simulink model "AVIC_model"  (R2015b)
settings: Solver=ode45  StartTime=0.0  StopTime=simtime  RelTol=1e-3
values from neighbouring files (symbols this model uses):
  A = 1    [simulation.m]
  a1 = 1    [simulation.m]
  a2 = 3    [simulation.m]
  a3 = 3    [simulation.m]
  Amp1 = Ampl/1000000    (= 134.217728)    [simulation.m]
  b1 = 1    [simulation.m]
  B2 = 8    [simulation.m]
  C = 32    [simulation.m]
  c1 = 1    [simulation.m]
  c2 = 1    [simulation.m]
  c3 = 1    [simulation.m]
  finrad = 2*pi/(N)*f0*clk    [simulation.m]
  FSC = 2^27    (= 134217728)    [simulation.m]
  SAT = 127    [simulation.m]
  Ts = 1/clk    (= 1.62760416667e-07)    [simulation.m]
libraries: simulink x298
(part 3 of 5)

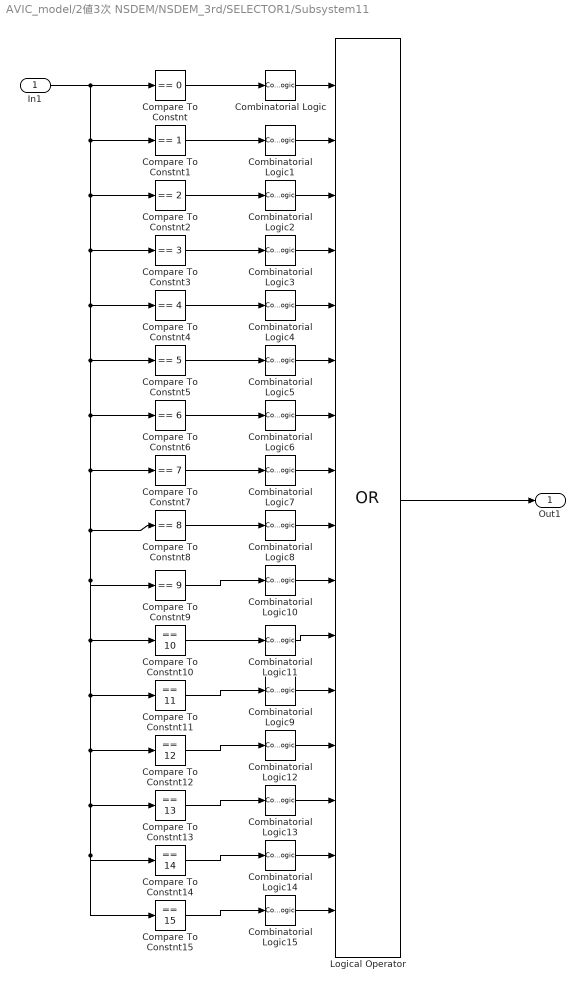
== system AVIC_model/2値3次 NSDEM/NSDEM_3rd/SELECTOR1/Subsystem11 ==
  In1 : Inport
  Combinatorial Logic : CombinatorialLogic  TruthTable=[0 0 0 0 0 0 0 0 0 0 0 0 0 0 0 0;1 0 0 0 0 0 0 0 0 0 0 0 0 0 0 0]
  Combinatorial Logic1 : CombinatorialLogic  TruthTable=[0 0 0 0 0 0 0 0 0 0 0 0 0 0 0 0; 0 1 0 0 0 0 0 0 0 0 0 0 0 0 0 0]
  Combinatorial Logic10 : CombinatorialLogic  TruthTable=[0 0 0 0 0 0 0 0 0 0 0 0 0 0 0 0;0 0 0 0 0 0 0 0 0 1 0 0 0 0 0 0]
  Combinatorial Logic11 : CombinatorialLogic  TruthTable=[0 0 0 0 0 0 0 0 0 0 0 0 0 0 0 0;0 0 0 0 0 0 0 0 0 0 1 0 0 0 0 0 ]
  Combinatorial Logic12 : CombinatorialLogic  TruthTable=[0 0 0 0 0 0 0 0 0 0 0 0 0 0 0 0;0 0 0 0 0 0 0 0 0 0 0 0 1 0 0 0]
  Combinatorial Logic13 : CombinatorialLogic  TruthTable=[0 0 0 0 0 0 0 0 0 0 0 0 0 0 0 0;0 0 0 0 0 0 0 0 0 0 0 0 0 1 0 0]
  Combinatorial Logic14 : CombinatorialLogic  TruthTable=[0 0 0 0 0 0 0 0 0 0 0 0 0 0 0 0;0 0 0 0 0 0 0 0 0 0 0 0 0 0 1 0]
  Combinatorial Logic15 : CombinatorialLogic  TruthTable=[0 0 0 0 0 0 0 0 0 0 0 0 0 0 0 0;0 0 0 0 0 0 0 0 0 0 0 0 0 0 0 1]
  Combinatorial Logic2 : CombinatorialLogic  TruthTable=[0 0 0 0 0 0 0 0 0 0 0 0 0 0 0 0;0 0 1 0 0 0 0 0 0 0 0 0 0 0 0 0]
  Combinatorial Logic3 : CombinatorialLogic  TruthTable=[0 0 0 0 0 0 0 0 0 0 0 0 0 0 0 0;0 0 0 1 0 0 0 0 0 0 0 0 0 0 0 0]
  Combinatorial Logic4 : CombinatorialLogic  TruthTable=[0 0 0 0 0 0 0 0 0 0 0 0 0 0 0 0;0 0 0 0 1 0 0 0 0 0 0 0 0 0 0 0]
  Combinatorial Logic5 : CombinatorialLogic  TruthTable=[0 0 0 0 0 0 0 0 0 0 0 0 0 0 0 0;0 0 0 0 0 1 0 0 0 0 0 0 0 0 0 0]
  Combinatorial Logic6 : CombinatorialLogic  TruthTable=[0 0 0 0 0 0 0 0 0 0 0 0 0 0 0 0;0 0 0 0 0 0 1 0 0 0 0 0 0 0 0 0]
  Combinatorial Logic7 : CombinatorialLogic  TruthTable=[0 0 0 0 0 0 0 0 0 0 0 0 0 0 0 0;0 0 0 0 0 0 0 1 0 0 0 0 0 0 0 0]
  Combinatorial Logic8 : CombinatorialLogic  TruthTable=[0 0 0 0 0 0 0 0 0 0 0 0 0 0 0 0;0 0 0 0 0 0 0 0 1 0 0 0 0 0 0 0]
  Combinatorial Logic9 : CombinatorialLogic  TruthTable=[0 0 0 0 0 0 0 0 0 0 0 0 0 0 0 0;0 0 0 0 0 0 0 0 0 0 0 1 0 0 0 0 ]
  Compare To Constnt : simulink/Logic and Bit Operations/Compare To Constant  relop===  const=0  OutDataTypeStr=boolean  ZeroCross=off
  Compare To Constnt1 : simulink/Logic and Bit Operations/Compare To Constant  relop===  const=1  OutDataTypeStr=boolean  ZeroCross=off
  Compare To Constnt10 : simulink/Logic and Bit Operations/Compare To Constant  relop===  const=10  OutDataTypeStr=boolean  ZeroCross=off
  Compare To Constnt11 : simulink/Logic and Bit Operations/Compare To Constant  relop===  const=11  OutDataTypeStr=boolean  ZeroCross=off
  Compare To Constnt12 : simulink/Logic and Bit Operations/Compare To Constant  relop===  const=12  OutDataTypeStr=boolean  ZeroCross=off
  Compare To Constnt13 : simulink/Logic and Bit Operations/Compare To Constant  relop===  const=13  OutDataTypeStr=boolean  ZeroCross=off
  Compare To Constnt14 : simulink/Logic and Bit Operations/Compare To Constant  relop===  const=14  OutDataTypeStr=boolean  ZeroCross=off
  Compare To Constnt15 : simulink/Logic and Bit Operations/Compare To Constant  relop===  const=15  OutDataTypeStr=boolean  ZeroCross=off
  Compare To Constnt2 : simulink/Logic and Bit Operations/Compare To Constant  relop===  const=2  OutDataTypeStr=boolean  ZeroCross=off
  Compare To Constnt3 : simulink/Logic and Bit Operations/Compare To Constant  relop===  const=3  OutDataTypeStr=boolean  ZeroCross=off
  Compare To Constnt4 : simulink/Logic and Bit Operations/Compare To Constant  relop===  const=4  OutDataTypeStr=boolean  ZeroCross=off
  Compare To Constnt5 : simulink/Logic and Bit Operations/Compare To Constant  relop===  const=5  OutDataTypeStr=boolean  ZeroCross=off
  Compare To Constnt6 : simulink/Logic and Bit Operations/Compare To Constant  relop===  const=6  OutDataTypeStr=boolean  ZeroCross=off
  Compare To Constnt7 : simulink/Logic and Bit Operations/Compare To Constant  relop===  const=7  OutDataTypeStr=boolean  ZeroCross=off
  Compare To Constnt8 : simulink/Logic and Bit Operations/Compare To Constant  relop===  const=8  OutDataTypeStr=boolean  ZeroCross=off
  Compare To Constnt9 : simulink/Logic and Bit Operations/Compare To Constant  relop===  const=9  OutDataTypeStr=boolean  ZeroCross=off
  Logical Operator : Logic  Operator=OR  Inputs=16  AllPortsSameDT=off  OutDataTypeStr=boolean
  Out1 : Outport
  wires:
  Logical Operator/1 -> Out1/1
  In1/1 -> Compare To Constnt/1, Compare To Constnt1/1, Compare To Constnt2/1, Compare To Constnt3/1, Compare To Constnt4/1, Compare To Constnt5/1, Compare To Constnt6/1, Compare To Constnt7/1, Compare To Constnt8/1, Compare To Constnt9/1, Compare To Constnt10/1, Compare To Constnt11/1, Compare To Constnt12/1, Compare To Constnt13/1, Compare To Constnt15/1, Compare To Constnt14/1
  Compare To Constnt/1 -> Combinatorial Logic/1
  Compare To Constnt1/1 -> Combinatorial Logic1/1
  Compare To Constnt2/1 -> Combinatorial Logic2/1
  Compare To Constnt3/1 -> Combinatorial Logic3/1
  Compare To Constnt4/1 -> Combinatorial Logic4/1
  Compare To Constnt5/1 -> Combinatorial Logic5/1
  Compare To Constnt6/1 -> Combinatorial Logic6/1
  Compare To Constnt7/1 -> Combinatorial Logic7/1
  Combinatorial Logic/1 -> Logical Operator/1
  Combinatorial Logic1/1 -> Logical Operator/2
  Combinatorial Logic2/1 -> Logical Operator/3
  Combinatorial Logic3/1 -> Logical Operator/4
  Combinatorial Logic4/1 -> Logical Operator/5
  Combinatorial Logic5/1 -> Logical Operator/6
  Combinatorial Logic6/1 -> Logical Operator/7
  Combinatorial Logic7/1 -> Logical Operator/8
  Compare To Constnt8/1 -> Combinatorial Logic8/1
  Compare To Constnt9/1 -> Combinatorial Logic10/1
  Compare To Constnt10/1 -> Combinatorial Logic11/1
  Compare To Constnt11/1 -> Combinatorial Logic9/1
  Compare To Constnt12/1 -> Combinatorial Logic12/1
  Compare To Constnt13/1 -> Combinatorial Logic13/1
  Compare To Constnt14/1 -> Combinatorial Logic14/1
  Compare To Constnt15/1 -> Combinatorial Logic15/1
  Combinatorial Logic8/1 -> Logical Operator/9
  Combinatorial Logic10/1 -> Logical Operator/10
  Combinatorial Logic11/1 -> Logical Operator/11
  Combinatorial Logic9/1 -> Logical Operator/12
  Combinatorial Logic12/1 -> Logical Operator/13
  Combinatorial Logic13/1 -> Logical Operator/14
  Combinatorial Logic14/1 -> Logical Operator/15
  Combinatorial Logic15/1 -> Logical Operator/16

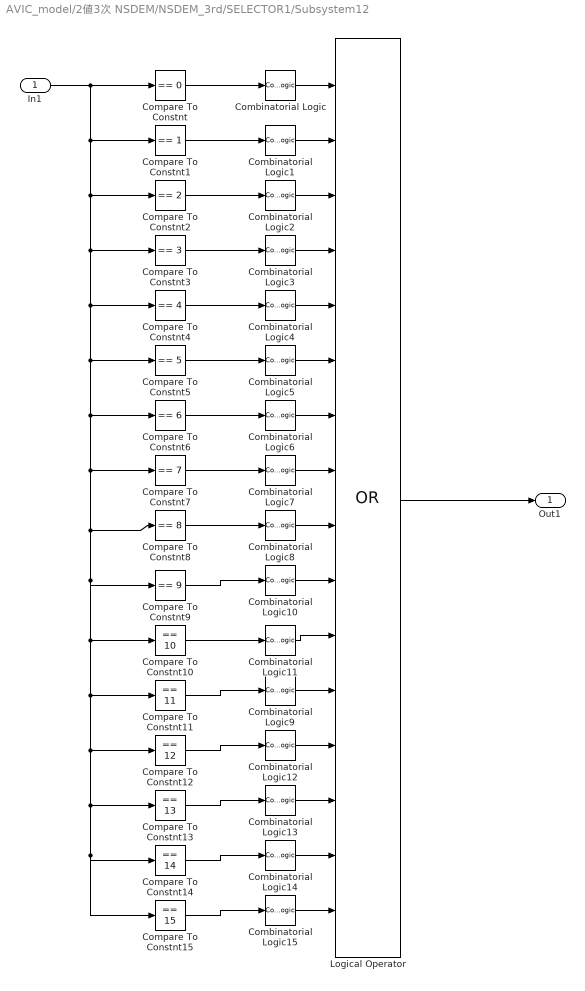
== system AVIC_model/2値3次 NSDEM/NSDEM_3rd/SELECTOR1/Subsystem12 ==
  In1 : Inport
  Combinatorial Logic : CombinatorialLogic  TruthTable=[0 0 0 0 0 0 0 0 0 0 0 0 0 0 0 0;1 0 0 0 0 0 0 0 0 0 0 0 0 0 0 0]
  Combinatorial Logic1 : CombinatorialLogic  TruthTable=[0 0 0 0 0 0 0 0 0 0 0 0 0 0 0 0; 0 1 0 0 0 0 0 0 0 0 0 0 0 0 0 0]
  Combinatorial Logic10 : CombinatorialLogic  TruthTable=[0 0 0 0 0 0 0 0 0 0 0 0 0 0 0 0;0 0 0 0 0 0 0 0 0 1 0 0 0 0 0 0]
  Combinatorial Logic11 : CombinatorialLogic  TruthTable=[0 0 0 0 0 0 0 0 0 0 0 0 0 0 0 0;0 0 0 0 0 0 0 0 0 0 1 0 0 0 0 0 ]
  Combinatorial Logic12 : CombinatorialLogic  TruthTable=[0 0 0 0 0 0 0 0 0 0 0 0 0 0 0 0;0 0 0 0 0 0 0 0 0 0 0 0 1 0 0 0]
  Combinatorial Logic13 : CombinatorialLogic  TruthTable=[0 0 0 0 0 0 0 0 0 0 0 0 0 0 0 0;0 0 0 0 0 0 0 0 0 0 0 0 0 1 0 0]
  Combinatorial Logic14 : CombinatorialLogic  TruthTable=[0 0 0 0 0 0 0 0 0 0 0 0 0 0 0 0;0 0 0 0 0 0 0 0 0 0 0 0 0 0 1 0]
  Combinatorial Logic15 : CombinatorialLogic  TruthTable=[0 0 0 0 0 0 0 0 0 0 0 0 0 0 0 0;0 0 0 0 0 0 0 0 0 0 0 0 0 0 0 1]
  Combinatorial Logic2 : CombinatorialLogic  TruthTable=[0 0 0 0 0 0 0 0 0 0 0 0 0 0 0 0;0 0 1 0 0 0 0 0 0 0 0 0 0 0 0 0]
  Combinatorial Logic3 : CombinatorialLogic  TruthTable=[0 0 0 0 0 0 0 0 0 0 0 0 0 0 0 0;0 0 0 1 0 0 0 0 0 0 0 0 0 0 0 0]
  Combinatorial Logic4 : CombinatorialLogic  TruthTable=[0 0 0 0 0 0 0 0 0 0 0 0 0 0 0 0;0 0 0 0 1 0 0 0 0 0 0 0 0 0 0 0]
  Combinatorial Logic5 : CombinatorialLogic  TruthTable=[0 0 0 0 0 0 0 0 0 0 0 0 0 0 0 0;0 0 0 0 0 1 0 0 0 0 0 0 0 0 0 0]
  Combinatorial Logic6 : CombinatorialLogic  TruthTable=[0 0 0 0 0 0 0 0 0 0 0 0 0 0 0 0;0 0 0 0 0 0 1 0 0 0 0 0 0 0 0 0]
  Combinatorial Logic7 : CombinatorialLogic  TruthTable=[0 0 0 0 0 0 0 0 0 0 0 0 0 0 0 0;0 0 0 0 0 0 0 1 0 0 0 0 0 0 0 0]
  Combinatorial Logic8 : CombinatorialLogic  TruthTable=[0 0 0 0 0 0 0 0 0 0 0 0 0 0 0 0;0 0 0 0 0 0 0 0 1 0 0 0 0 0 0 0]
  Combinatorial Logic9 : CombinatorialLogic  TruthTable=[0 0 0 0 0 0 0 0 0 0 0 0 0 0 0 0;0 0 0 0 0 0 0 0 0 0 0 1 0 0 0 0 ]
  Compare To Constnt : simulink/Logic and Bit Operations/Compare To Constant  relop===  const=0  OutDataTypeStr=boolean  ZeroCross=off
  Compare To Constnt1 : simulink/Logic and Bit Operations/Compare To Constant  relop===  const=1  OutDataTypeStr=boolean  ZeroCross=off
  Compare To Constnt10 : simulink/Logic and Bit Operations/Compare To Constant  relop===  const=10  OutDataTypeStr=boolean  ZeroCross=off
  Compare To Constnt11 : simulink/Logic and Bit Operations/Compare To Constant  relop===  const=11  OutDataTypeStr=boolean  ZeroCross=off
  Compare To Constnt12 : simulink/Logic and Bit Operations/Compare To Constant  relop===  const=12  OutDataTypeStr=boolean  ZeroCross=off
  Compare To Constnt13 : simulink/Logic and Bit Operations/Compare To Constant  relop===  const=13  OutDataTypeStr=boolean  ZeroCross=off
  Compare To Constnt14 : simulink/Logic and Bit Operations/Compare To Constant  relop===  const=14  OutDataTypeStr=boolean  ZeroCross=off
  Compare To Constnt15 : simulink/Logic and Bit Operations/Compare To Constant  relop===  const=15  OutDataTypeStr=boolean  ZeroCross=off
  Compare To Constnt2 : simulink/Logic and Bit Operations/Compare To Constant  relop===  const=2  OutDataTypeStr=boolean  ZeroCross=off
  Compare To Constnt3 : simulink/Logic and Bit Operations/Compare To Constant  relop===  const=3  OutDataTypeStr=boolean  ZeroCross=off
  Compare To Constnt4 : simulink/Logic and Bit Operations/Compare To Constant  relop===  const=4  OutDataTypeStr=boolean  ZeroCross=off
  Compare To Constnt5 : simulink/Logic and Bit Operations/Compare To Constant  relop===  const=5  OutDataTypeStr=boolean  ZeroCross=off
  Compare To Constnt6 : simulink/Logic and Bit Operations/Compare To Constant  relop===  const=6  OutDataTypeStr=boolean  ZeroCross=off
  Compare To Constnt7 : simulink/Logic and Bit Operations/Compare To Constant  relop===  const=7  OutDataTypeStr=boolean  ZeroCross=off
  Compare To Constnt8 : simulink/Logic and Bit Operations/Compare To Constant  relop===  const=8  OutDataTypeStr=boolean  ZeroCross=off
  Compare To Constnt9 : simulink/Logic and Bit Operations/Compare To Constant  relop===  const=9  OutDataTypeStr=boolean  ZeroCross=off
  Logical Operator : Logic  Operator=OR  Inputs=16  AllPortsSameDT=off  OutDataTypeStr=boolean
  Out1 : Outport
  wires:
  Logical Operator/1 -> Out1/1
  In1/1 -> Compare To Constnt/1, Compare To Constnt1/1, Compare To Constnt2/1, Compare To Constnt3/1, Compare To Constnt4/1, Compare To Constnt5/1, Compare To Constnt6/1, Compare To Constnt7/1, Compare To Constnt8/1, Compare To Constnt9/1, Compare To Constnt10/1, Compare To Constnt11/1, Compare To Constnt12/1, Compare To Constnt13/1, Compare To Constnt15/1, Compare To Constnt14/1
  Compare To Constnt/1 -> Combinatorial Logic/1
  Compare To Constnt1/1 -> Combinatorial Logic1/1
  Compare To Constnt2/1 -> Combinatorial Logic2/1
  Compare To Constnt3/1 -> Combinatorial Logic3/1
  Compare To Constnt4/1 -> Combinatorial Logic4/1
  Compare To Constnt5/1 -> Combinatorial Logic5/1
  Compare To Constnt6/1 -> Combinatorial Logic6/1
  Compare To Constnt7/1 -> Combinatorial Logic7/1
  Combinatorial Logic/1 -> Logical Operator/1
  Combinatorial Logic1/1 -> Logical Operator/2
  Combinatorial Logic2/1 -> Logical Operator/3
  Combinatorial Logic3/1 -> Logical Operator/4
  Combinatorial Logic4/1 -> Logical Operator/5
  Combinatorial Logic5/1 -> Logical Operator/6
  Combinatorial Logic6/1 -> Logical Operator/7
  Combinatorial Logic7/1 -> Logical Operator/8
  Compare To Constnt8/1 -> Combinatorial Logic8/1
  Compare To Constnt9/1 -> Combinatorial Logic10/1
  Compare To Constnt10/1 -> Combinatorial Logic11/1
  Compare To Constnt11/1 -> Combinatorial Logic9/1
  Compare To Constnt12/1 -> Combinatorial Logic12/1
  Compare To Constnt13/1 -> Combinatorial Logic13/1
  Compare To Constnt14/1 -> Combinatorial Logic14/1
  Compare To Constnt15/1 -> Combinatorial Logic15/1
  Combinatorial Logic8/1 -> Logical Operator/9
  Combinatorial Logic10/1 -> Logical Operator/10
  Combinatorial Logic11/1 -> Logical Operator/11
  Combinatorial Logic9/1 -> Logical Operator/12
  Combinatorial Logic12/1 -> Logical Operator/13
  Combinatorial Logic13/1 -> Logical Operator/14
  Combinatorial Logic14/1 -> Logical Operator/15
  Combinatorial Logic15/1 -> Logical Operator/16

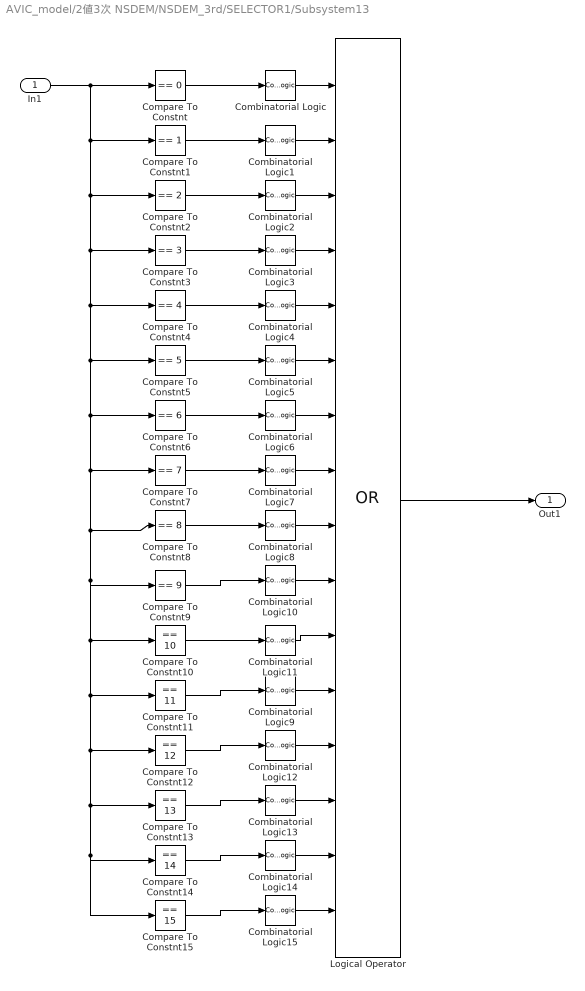
== system AVIC_model/2値3次 NSDEM/NSDEM_3rd/SELECTOR1/Subsystem13 ==
  In1 : Inport
  Combinatorial Logic : CombinatorialLogic  TruthTable=[0 0 0 0 0 0 0 0 0 0 0 0 0 0 0 0;1 0 0 0 0 0 0 0 0 0 0 0 0 0 0 0]
  Combinatorial Logic1 : CombinatorialLogic  TruthTable=[0 0 0 0 0 0 0 0 0 0 0 0 0 0 0 0; 0 1 0 0 0 0 0 0 0 0 0 0 0 0 0 0]
  Combinatorial Logic10 : CombinatorialLogic  TruthTable=[0 0 0 0 0 0 0 0 0 0 0 0 0 0 0 0;0 0 0 0 0 0 0 0 0 1 0 0 0 0 0 0]
  Combinatorial Logic11 : CombinatorialLogic  TruthTable=[0 0 0 0 0 0 0 0 0 0 0 0 0 0 0 0;0 0 0 0 0 0 0 0 0 0 1 0 0 0 0 0 ]
  Combinatorial Logic12 : CombinatorialLogic  TruthTable=[0 0 0 0 0 0 0 0 0 0 0 0 0 0 0 0;0 0 0 0 0 0 0 0 0 0 0 0 1 0 0 0]
  Combinatorial Logic13 : CombinatorialLogic  TruthTable=[0 0 0 0 0 0 0 0 0 0 0 0 0 0 0 0;0 0 0 0 0 0 0 0 0 0 0 0 0 1 0 0]
  Combinatorial Logic14 : CombinatorialLogic  TruthTable=[0 0 0 0 0 0 0 0 0 0 0 0 0 0 0 0;0 0 0 0 0 0 0 0 0 0 0 0 0 0 1 0]
  Combinatorial Logic15 : CombinatorialLogic  TruthTable=[0 0 0 0 0 0 0 0 0 0 0 0 0 0 0 0;0 0 0 0 0 0 0 0 0 0 0 0 0 0 0 1]
  Combinatorial Logic2 : CombinatorialLogic  TruthTable=[0 0 0 0 0 0 0 0 0 0 0 0 0 0 0 0;0 0 1 0 0 0 0 0 0 0 0 0 0 0 0 0]
  Combinatorial Logic3 : CombinatorialLogic  TruthTable=[0 0 0 0 0 0 0 0 0 0 0 0 0 0 0 0;0 0 0 1 0 0 0 0 0 0 0 0 0 0 0 0]
  Combinatorial Logic4 : CombinatorialLogic  TruthTable=[0 0 0 0 0 0 0 0 0 0 0 0 0 0 0 0;0 0 0 0 1 0 0 0 0 0 0 0 0 0 0 0]
  Combinatorial Logic5 : CombinatorialLogic  TruthTable=[0 0 0 0 0 0 0 0 0 0 0 0 0 0 0 0;0 0 0 0 0 1 0 0 0 0 0 0 0 0 0 0]
  Combinatorial Logic6 : CombinatorialLogic  TruthTable=[0 0 0 0 0 0 0 0 0 0 0 0 0 0 0 0;0 0 0 0 0 0 1 0 0 0 0 0 0 0 0 0]
  Combinatorial Logic7 : CombinatorialLogic  TruthTable=[0 0 0 0 0 0 0 0 0 0 0 0 0 0 0 0;0 0 0 0 0 0 0 1 0 0 0 0 0 0 0 0]
  Combinatorial Logic8 : CombinatorialLogic  TruthTable=[0 0 0 0 0 0 0 0 0 0 0 0 0 0 0 0;0 0 0 0 0 0 0 0 1 0 0 0 0 0 0 0]
  Combinatorial Logic9 : CombinatorialLogic  TruthTable=[0 0 0 0 0 0 0 0 0 0 0 0 0 0 0 0;0 0 0 0 0 0 0 0 0 0 0 1 0 0 0 0 ]
  Compare To Constnt : simulink/Logic and Bit Operations/Compare To Constant  relop===  const=0  OutDataTypeStr=boolean  ZeroCross=off
  Compare To Constnt1 : simulink/Logic and Bit Operations/Compare To Constant  relop===  const=1  OutDataTypeStr=boolean  ZeroCross=off
  Compare To Constnt10 : simulink/Logic and Bit Operations/Compare To Constant  relop===  const=10  OutDataTypeStr=boolean  ZeroCross=off
  Compare To Constnt11 : simulink/Logic and Bit Operations/Compare To Constant  relop===  const=11  OutDataTypeStr=boolean  ZeroCross=off
  Compare To Constnt12 : simulink/Logic and Bit Operations/Compare To Constant  relop===  const=12  OutDataTypeStr=boolean  ZeroCross=off
  Compare To Constnt13 : simulink/Logic and Bit Operations/Compare To Constant  relop===  const=13  OutDataTypeStr=boolean  ZeroCross=off
  Compare To Constnt14 : simulink/Logic and Bit Operations/Compare To Constant  relop===  const=14  OutDataTypeStr=boolean  ZeroCross=off
  Compare To Constnt15 : simulink/Logic and Bit Operations/Compare To Constant  relop===  const=15  OutDataTypeStr=boolean  ZeroCross=off
  Compare To Constnt2 : simulink/Logic and Bit Operations/Compare To Constant  relop===  const=2  OutDataTypeStr=boolean  ZeroCross=off
  Compare To Constnt3 : simulink/Logic and Bit Operations/Compare To Constant  relop===  const=3  OutDataTypeStr=boolean  ZeroCross=off
  Compare To Constnt4 : simulink/Logic and Bit Operations/Compare To Constant  relop===  const=4  OutDataTypeStr=boolean  ZeroCross=off
  Compare To Constnt5 : simulink/Logic and Bit Operations/Compare To Constant  relop===  const=5  OutDataTypeStr=boolean  ZeroCross=off
  Compare To Constnt6 : simulink/Logic and Bit Operations/Compare To Constant  relop===  const=6  OutDataTypeStr=boolean  ZeroCross=off
  Compare To Constnt7 : simulink/Logic and Bit Operations/Compare To Constant  relop===  const=7  OutDataTypeStr=boolean  ZeroCross=off
  Compare To Constnt8 : simulink/Logic and Bit Operations/Compare To Constant  relop===  const=8  OutDataTypeStr=boolean  ZeroCross=off
  Compare To Constnt9 : simulink/Logic and Bit Operations/Compare To Constant  relop===  const=9  OutDataTypeStr=boolean  ZeroCross=off
  Logical Operator : Logic  Operator=OR  Inputs=16  AllPortsSameDT=off  OutDataTypeStr=boolean
  Out1 : Outport
  wires:
  Logical Operator/1 -> Out1/1
  In1/1 -> Compare To Constnt/1, Compare To Constnt1/1, Compare To Constnt2/1, Compare To Constnt3/1, Compare To Constnt4/1, Compare To Constnt5/1, Compare To Constnt6/1, Compare To Constnt7/1, Compare To Constnt8/1, Compare To Constnt9/1, Compare To Constnt10/1, Compare To Constnt11/1, Compare To Constnt12/1, Compare To Constnt13/1, Compare To Constnt15/1, Compare To Constnt14/1
  Compare To Constnt/1 -> Combinatorial Logic/1
  Compare To Constnt1/1 -> Combinatorial Logic1/1
  Compare To Constnt2/1 -> Combinatorial Logic2/1
  Compare To Constnt3/1 -> Combinatorial Logic3/1
  Compare To Constnt4/1 -> Combinatorial Logic4/1
  Compare To Constnt5/1 -> Combinatorial Logic5/1
  Compare To Constnt6/1 -> Combinatorial Logic6/1
  Compare To Constnt7/1 -> Combinatorial Logic7/1
  Combinatorial Logic/1 -> Logical Operator/1
  Combinatorial Logic1/1 -> Logical Operator/2
  Combinatorial Logic2/1 -> Logical Operator/3
  Combinatorial Logic3/1 -> Logical Operator/4
  Combinatorial Logic4/1 -> Logical Operator/5
  Combinatorial Logic5/1 -> Logical Operator/6
  Combinatorial Logic6/1 -> Logical Operator/7
  Combinatorial Logic7/1 -> Logical Operator/8
  Compare To Constnt8/1 -> Combinatorial Logic8/1
  Compare To Constnt9/1 -> Combinatorial Logic10/1
  Compare To Constnt10/1 -> Combinatorial Logic11/1
  Compare To Constnt11/1 -> Combinatorial Logic9/1
  Compare To Constnt12/1 -> Combinatorial Logic12/1
  Compare To Constnt13/1 -> Combinatorial Logic13/1
  Compare To Constnt14/1 -> Combinatorial Logic14/1
  Compare To Constnt15/1 -> Combinatorial Logic15/1
  Combinatorial Logic8/1 -> Logical Operator/9
  Combinatorial Logic10/1 -> Logical Operator/10
  Combinatorial Logic11/1 -> Logical Operator/11
  Combinatorial Logic9/1 -> Logical Operator/12
  Combinatorial Logic12/1 -> Logical Operator/13
  Combinatorial Logic13/1 -> Logical Operator/14
  Combinatorial Logic14/1 -> Logical Operator/15
  Combinatorial Logic15/1 -> Logical Operator/16

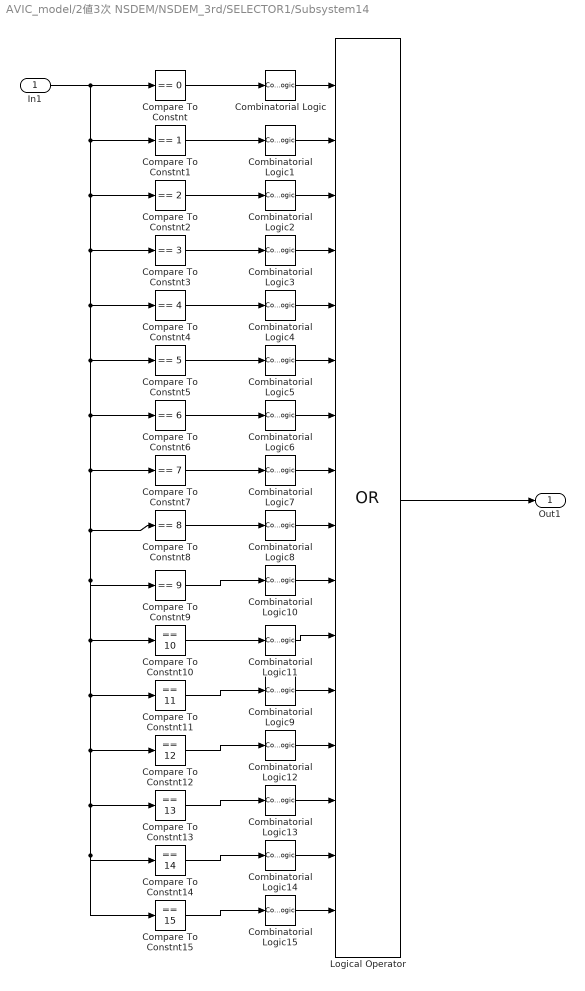
== system AVIC_model/2値3次 NSDEM/NSDEM_3rd/SELECTOR1/Subsystem14 ==
  In1 : Inport
  Combinatorial Logic : CombinatorialLogic  TruthTable=[0 0 0 0 0 0 0 0 0 0 0 0 0 0 0 0;1 0 0 0 0 0 0 0 0 0 0 0 0 0 0 0]
  Combinatorial Logic1 : CombinatorialLogic  TruthTable=[0 0 0 0 0 0 0 0 0 0 0 0 0 0 0 0; 0 1 0 0 0 0 0 0 0 0 0 0 0 0 0 0]
  Combinatorial Logic10 : CombinatorialLogic  TruthTable=[0 0 0 0 0 0 0 0 0 0 0 0 0 0 0 0;0 0 0 0 0 0 0 0 0 1 0 0 0 0 0 0]
  Combinatorial Logic11 : CombinatorialLogic  TruthTable=[0 0 0 0 0 0 0 0 0 0 0 0 0 0 0 0;0 0 0 0 0 0 0 0 0 0 1 0 0 0 0 0 ]
  Combinatorial Logic12 : CombinatorialLogic  TruthTable=[0 0 0 0 0 0 0 0 0 0 0 0 0 0 0 0;0 0 0 0 0 0 0 0 0 0 0 0 1 0 0 0]
  Combinatorial Logic13 : CombinatorialLogic  TruthTable=[0 0 0 0 0 0 0 0 0 0 0 0 0 0 0 0;0 0 0 0 0 0 0 0 0 0 0 0 0 1 0 0]
  Combinatorial Logic14 : CombinatorialLogic  TruthTable=[0 0 0 0 0 0 0 0 0 0 0 0 0 0 0 0;0 0 0 0 0 0 0 0 0 0 0 0 0 0 1 0]
  Combinatorial Logic15 : CombinatorialLogic  TruthTable=[0 0 0 0 0 0 0 0 0 0 0 0 0 0 0 0;0 0 0 0 0 0 0 0 0 0 0 0 0 0 0 1]
  Combinatorial Logic2 : CombinatorialLogic  TruthTable=[0 0 0 0 0 0 0 0 0 0 0 0 0 0 0 0;0 0 1 0 0 0 0 0 0 0 0 0 0 0 0 0]
  Combinatorial Logic3 : CombinatorialLogic  TruthTable=[0 0 0 0 0 0 0 0 0 0 0 0 0 0 0 0;0 0 0 1 0 0 0 0 0 0 0 0 0 0 0 0]
  Combinatorial Logic4 : CombinatorialLogic  TruthTable=[0 0 0 0 0 0 0 0 0 0 0 0 0 0 0 0;0 0 0 0 1 0 0 0 0 0 0 0 0 0 0 0]
  Combinatorial Logic5 : CombinatorialLogic  TruthTable=[0 0 0 0 0 0 0 0 0 0 0 0 0 0 0 0;0 0 0 0 0 1 0 0 0 0 0 0 0 0 0 0]
  Combinatorial Logic6 : CombinatorialLogic  TruthTable=[0 0 0 0 0 0 0 0 0 0 0 0 0 0 0 0;0 0 0 0 0 0 1 0 0 0 0 0 0 0 0 0]
  Combinatorial Logic7 : CombinatorialLogic  TruthTable=[0 0 0 0 0 0 0 0 0 0 0 0 0 0 0 0;0 0 0 0 0 0 0 1 0 0 0 0 0 0 0 0]
  Combinatorial Logic8 : CombinatorialLogic  TruthTable=[0 0 0 0 0 0 0 0 0 0 0 0 0 0 0 0;0 0 0 0 0 0 0 0 1 0 0 0 0 0 0 0]
  Combinatorial Logic9 : CombinatorialLogic  TruthTable=[0 0 0 0 0 0 0 0 0 0 0 0 0 0 0 0;0 0 0 0 0 0 0 0 0 0 0 1 0 0 0 0 ]
  Compare To Constnt : simulink/Logic and Bit Operations/Compare To Constant  relop===  const=0  OutDataTypeStr=boolean  ZeroCross=off
  Compare To Constnt1 : simulink/Logic and Bit Operations/Compare To Constant  relop===  const=1  OutDataTypeStr=boolean  ZeroCross=off
  Compare To Constnt10 : simulink/Logic and Bit Operations/Compare To Constant  relop===  const=10  OutDataTypeStr=boolean  ZeroCross=off
  Compare To Constnt11 : simulink/Logic and Bit Operations/Compare To Constant  relop===  const=11  OutDataTypeStr=boolean  ZeroCross=off
  Compare To Constnt12 : simulink/Logic and Bit Operations/Compare To Constant  relop===  const=12  OutDataTypeStr=boolean  ZeroCross=off
  Compare To Constnt13 : simulink/Logic and Bit Operations/Compare To Constant  relop===  const=13  OutDataTypeStr=boolean  ZeroCross=off
  Compare To Constnt14 : simulink/Logic and Bit Operations/Compare To Constant  relop===  const=14  OutDataTypeStr=boolean  ZeroCross=off
  Compare To Constnt15 : simulink/Logic and Bit Operations/Compare To Constant  relop===  const=15  OutDataTypeStr=boolean  ZeroCross=off
  Compare To Constnt2 : simulink/Logic and Bit Operations/Compare To Constant  relop===  const=2  OutDataTypeStr=boolean  ZeroCross=off
  Compare To Constnt3 : simulink/Logic and Bit Operations/Compare To Constant  relop===  const=3  OutDataTypeStr=boolean  ZeroCross=off
  Compare To Constnt4 : simulink/Logic and Bit Operations/Compare To Constant  relop===  const=4  OutDataTypeStr=boolean  ZeroCross=off
  Compare To Constnt5 : simulink/Logic and Bit Operations/Compare To Constant  relop===  const=5  OutDataTypeStr=boolean  ZeroCross=off
  Compare To Constnt6 : simulink/Logic and Bit Operations/Compare To Constant  relop===  const=6  OutDataTypeStr=boolean  ZeroCross=off
  Compare To Constnt7 : simulink/Logic and Bit Operations/Compare To Constant  relop===  const=7  OutDataTypeStr=boolean  ZeroCross=off
  Compare To Constnt8 : simulink/Logic and Bit Operations/Compare To Constant  relop===  const=8  OutDataTypeStr=boolean  ZeroCross=off
  Compare To Constnt9 : simulink/Logic and Bit Operations/Compare To Constant  relop===  const=9  OutDataTypeStr=boolean  ZeroCross=off
  Logical Operator : Logic  Operator=OR  Inputs=16  AllPortsSameDT=off  OutDataTypeStr=boolean
  Out1 : Outport
  wires:
  Logical Operator/1 -> Out1/1
  In1/1 -> Compare To Constnt/1, Compare To Constnt1/1, Compare To Constnt2/1, Compare To Constnt3/1, Compare To Constnt4/1, Compare To Constnt5/1, Compare To Constnt6/1, Compare To Constnt7/1, Compare To Constnt8/1, Compare To Constnt9/1, Compare To Constnt10/1, Compare To Constnt11/1, Compare To Constnt12/1, Compare To Constnt13/1, Compare To Constnt15/1, Compare To Constnt14/1
  Compare To Constnt/1 -> Combinatorial Logic/1
  Compare To Constnt1/1 -> Combinatorial Logic1/1
  Compare To Constnt2/1 -> Combinatorial Logic2/1
  Compare To Constnt3/1 -> Combinatorial Logic3/1
  Compare To Constnt4/1 -> Combinatorial Logic4/1
  Compare To Constnt5/1 -> Combinatorial Logic5/1
  Compare To Constnt6/1 -> Combinatorial Logic6/1
  Compare To Constnt7/1 -> Combinatorial Logic7/1
  Combinatorial Logic/1 -> Logical Operator/1
  Combinatorial Logic1/1 -> Logical Operator/2
  Combinatorial Logic2/1 -> Logical Operator/3
  Combinatorial Logic3/1 -> Logical Operator/4
  Combinatorial Logic4/1 -> Logical Operator/5
  Combinatorial Logic5/1 -> Logical Operator/6
  Combinatorial Logic6/1 -> Logical Operator/7
  Combinatorial Logic7/1 -> Logical Operator/8
  Compare To Constnt8/1 -> Combinatorial Logic8/1
  Compare To Constnt9/1 -> Combinatorial Logic10/1
  Compare To Constnt10/1 -> Combinatorial Logic11/1
  Compare To Constnt11/1 -> Combinatorial Logic9/1
  Compare To Constnt12/1 -> Combinatorial Logic12/1
  Compare To Constnt13/1 -> Combinatorial Logic13/1
  Compare To Constnt14/1 -> Combinatorial Logic14/1
  Compare To Constnt15/1 -> Combinatorial Logic15/1
  Combinatorial Logic8/1 -> Logical Operator/9
  Combinatorial Logic10/1 -> Logical Operator/10
  Combinatorial Logic11/1 -> Logical Operator/11
  Combinatorial Logic9/1 -> Logical Operator/12
  Combinatorial Logic12/1 -> Logical Operator/13
  Combinatorial Logic13/1 -> Logical Operator/14
  Combinatorial Logic14/1 -> Logical Operator/15
  Combinatorial Logic15/1 -> Logical Operator/16

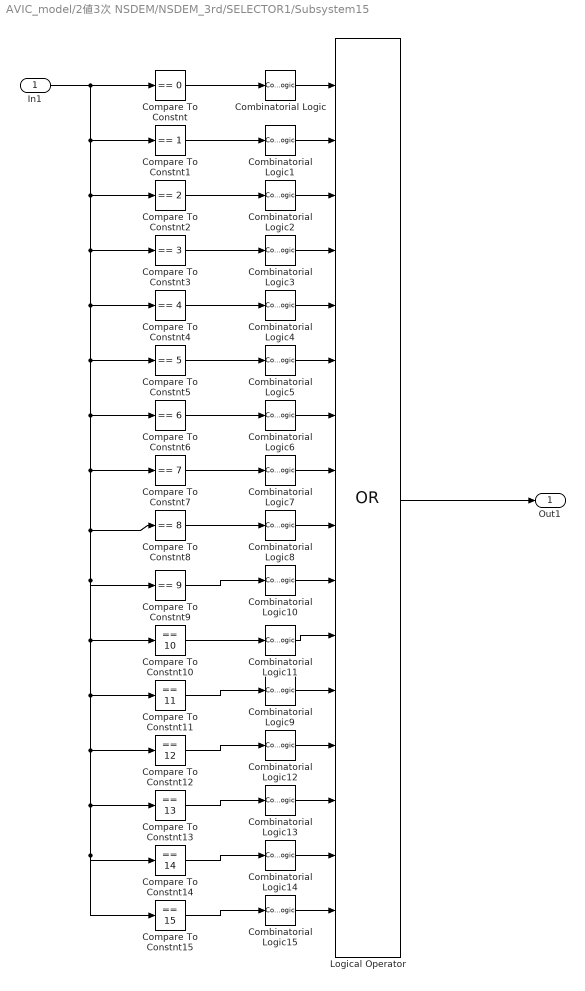
== system AVIC_model/2値3次 NSDEM/NSDEM_3rd/SELECTOR1/Subsystem15 ==
  In1 : Inport
  Combinatorial Logic : CombinatorialLogic  TruthTable=[0 0 0 0 0 0 0 0 0 0 0 0 0 0 0 0;1 0 0 0 0 0 0 0 0 0 0 0 0 0 0 0]
  Combinatorial Logic1 : CombinatorialLogic  TruthTable=[0 0 0 0 0 0 0 0 0 0 0 0 0 0 0 0; 0 1 0 0 0 0 0 0 0 0 0 0 0 0 0 0]
  Combinatorial Logic10 : CombinatorialLogic  TruthTable=[0 0 0 0 0 0 0 0 0 0 0 0 0 0 0 0;0 0 0 0 0 0 0 0 0 1 0 0 0 0 0 0]
  Combinatorial Logic11 : CombinatorialLogic  TruthTable=[0 0 0 0 0 0 0 0 0 0 0 0 0 0 0 0;0 0 0 0 0 0 0 0 0 0 1 0 0 0 0 0 ]
  Combinatorial Logic12 : CombinatorialLogic  TruthTable=[0 0 0 0 0 0 0 0 0 0 0 0 0 0 0 0;0 0 0 0 0 0 0 0 0 0 0 0 1 0 0 0]
  Combinatorial Logic13 : CombinatorialLogic  TruthTable=[0 0 0 0 0 0 0 0 0 0 0 0 0 0 0 0;0 0 0 0 0 0 0 0 0 0 0 0 0 1 0 0]
  Combinatorial Logic14 : CombinatorialLogic  TruthTable=[0 0 0 0 0 0 0 0 0 0 0 0 0 0 0 0;0 0 0 0 0 0 0 0 0 0 0 0 0 0 1 0]
  Combinatorial Logic15 : CombinatorialLogic  TruthTable=[0 0 0 0 0 0 0 0 0 0 0 0 0 0 0 0;0 0 0 0 0 0 0 0 0 0 0 0 0 0 0 1]
  Combinatorial Logic2 : CombinatorialLogic  TruthTable=[0 0 0 0 0 0 0 0 0 0 0 0 0 0 0 0;0 0 1 0 0 0 0 0 0 0 0 0 0 0 0 0]
  Combinatorial Logic3 : CombinatorialLogic  TruthTable=[0 0 0 0 0 0 0 0 0 0 0 0 0 0 0 0;0 0 0 1 0 0 0 0 0 0 0 0 0 0 0 0]
  Combinatorial Logic4 : CombinatorialLogic  TruthTable=[0 0 0 0 0 0 0 0 0 0 0 0 0 0 0 0;0 0 0 0 1 0 0 0 0 0 0 0 0 0 0 0]
  Combinatorial Logic5 : CombinatorialLogic  TruthTable=[0 0 0 0 0 0 0 0 0 0 0 0 0 0 0 0;0 0 0 0 0 1 0 0 0 0 0 0 0 0 0 0]
  Combinatorial Logic6 : CombinatorialLogic  TruthTable=[0 0 0 0 0 0 0 0 0 0 0 0 0 0 0 0;0 0 0 0 0 0 1 0 0 0 0 0 0 0 0 0]
  Combinatorial Logic7 : CombinatorialLogic  TruthTable=[0 0 0 0 0 0 0 0 0 0 0 0 0 0 0 0;0 0 0 0 0 0 0 1 0 0 0 0 0 0 0 0]
  Combinatorial Logic8 : CombinatorialLogic  TruthTable=[0 0 0 0 0 0 0 0 0 0 0 0 0 0 0 0;0 0 0 0 0 0 0 0 1 0 0 0 0 0 0 0]
  Combinatorial Logic9 : CombinatorialLogic  TruthTable=[0 0 0 0 0 0 0 0 0 0 0 0 0 0 0 0;0 0 0 0 0 0 0 0 0 0 0 1 0 0 0 0 ]
  Compare To Constnt : simulink/Logic and Bit Operations/Compare To Constant  relop===  const=0  OutDataTypeStr=boolean  ZeroCross=off
  Compare To Constnt1 : simulink/Logic and Bit Operations/Compare To Constant  relop===  const=1  OutDataTypeStr=boolean  ZeroCross=off
  Compare To Constnt10 : simulink/Logic and Bit Operations/Compare To Constant  relop===  const=10  OutDataTypeStr=boolean  ZeroCross=off
  Compare To Constnt11 : simulink/Logic and Bit Operations/Compare To Constant  relop===  const=11  OutDataTypeStr=boolean  ZeroCross=off
  Compare To Constnt12 : simulink/Logic and Bit Operations/Compare To Constant  relop===  const=12  OutDataTypeStr=boolean  ZeroCross=off
  Compare To Constnt13 : simulink/Logic and Bit Operations/Compare To Constant  relop===  const=13  OutDataTypeStr=boolean  ZeroCross=off
  Compare To Constnt14 : simulink/Logic and Bit Operations/Compare To Constant  relop===  const=14  OutDataTypeStr=boolean  ZeroCross=off
  Compare To Constnt15 : simulink/Logic and Bit Operations/Compare To Constant  relop===  const=15  OutDataTypeStr=boolean  ZeroCross=off
  Compare To Constnt2 : simulink/Logic and Bit Operations/Compare To Constant  relop===  const=2  OutDataTypeStr=boolean  ZeroCross=off
  Compare To Constnt3 : simulink/Logic and Bit Operations/Compare To Constant  relop===  const=3  OutDataTypeStr=boolean  ZeroCross=off
  Compare To Constnt4 : simulink/Logic and Bit Operations/Compare To Constant  relop===  const=4  OutDataTypeStr=boolean  ZeroCross=off
  Compare To Constnt5 : simulink/Logic and Bit Operations/Compare To Constant  relop===  const=5  OutDataTypeStr=boolean  ZeroCross=off
  Compare To Constnt6 : simulink/Logic and Bit Operations/Compare To Constant  relop===  const=6  OutDataTypeStr=boolean  ZeroCross=off
  Compare To Constnt7 : simulink/Logic and Bit Operations/Compare To Constant  relop===  const=7  OutDataTypeStr=boolean  ZeroCross=off
  Compare To Constnt8 : simulink/Logic and Bit Operations/Compare To Constant  relop===  const=8  OutDataTypeStr=boolean  ZeroCross=off
  Compare To Constnt9 : simulink/Logic and Bit Operations/Compare To Constant  relop===  const=9  OutDataTypeStr=boolean  ZeroCross=off
  Logical Operator : Logic  Operator=OR  Inputs=16  AllPortsSameDT=off  OutDataTypeStr=boolean
  Out1 : Outport
  wires:
  Logical Operator/1 -> Out1/1
  In1/1 -> Compare To Constnt/1, Compare To Constnt1/1, Compare To Constnt2/1, Compare To Constnt3/1, Compare To Constnt4/1, Compare To Constnt5/1, Compare To Constnt6/1, Compare To Constnt7/1, Compare To Constnt8/1, Compare To Constnt9/1, Compare To Constnt10/1, Compare To Constnt11/1, Compare To Constnt12/1, Compare To Constnt13/1, Compare To Constnt15/1, Compare To Constnt14/1
  Compare To Constnt/1 -> Combinatorial Logic/1
  Compare To Constnt1/1 -> Combinatorial Logic1/1
  Compare To Constnt2/1 -> Combinatorial Logic2/1
  Compare To Constnt3/1 -> Combinatorial Logic3/1
  Compare To Constnt4/1 -> Combinatorial Logic4/1
  Compare To Constnt5/1 -> Combinatorial Logic5/1
  Compare To Constnt6/1 -> Combinatorial Logic6/1
  Compare To Constnt7/1 -> Combinatorial Logic7/1
  Combinatorial Logic/1 -> Logical Operator/1
  Combinatorial Logic1/1 -> Logical Operator/2
  Combinatorial Logic2/1 -> Logical Operator/3
  Combinatorial Logic3/1 -> Logical Operator/4
  Combinatorial Logic4/1 -> Logical Operator/5
  Combinatorial Logic5/1 -> Logical Operator/6
  Combinatorial Logic6/1 -> Logical Operator/7
  Combinatorial Logic7/1 -> Logical Operator/8
  Compare To Constnt8/1 -> Combinatorial Logic8/1
  Compare To Constnt9/1 -> Combinatorial Logic10/1
  Compare To Constnt10/1 -> Combinatorial Logic11/1
  Compare To Constnt11/1 -> Combinatorial Logic9/1
  Compare To Constnt12/1 -> Combinatorial Logic12/1
  Compare To Constnt13/1 -> Combinatorial Logic13/1
  Compare To Constnt14/1 -> Combinatorial Logic14/1
  Compare To Constnt15/1 -> Combinatorial Logic15/1
  Combinatorial Logic8/1 -> Logical Operator/9
  Combinatorial Logic10/1 -> Logical Operator/10
  Combinatorial Logic11/1 -> Logical Operator/11
  Combinatorial Logic9/1 -> Logical Operator/12
  Combinatorial Logic12/1 -> Logical Operator/13
  Combinatorial Logic13/1 -> Logical Operator/14
  Combinatorial Logic14/1 -> Logical Operator/15
  Combinatorial Logic15/1 -> Logical Operator/16

== system AVIC_model/2値3次 NSDEM/NSDEM_3rd/SELECTOR1/Subsystem2 ==
  In1 : Inport
  Combinatorial Logic : CombinatorialLogic  TruthTable=[0 0 0 0 0 0 0 0 0 0 0 0 0 0 0 0;1 0 0 0 0 0 0 0 0 0 0 0 0 0 0 0]
  Combinatorial Logic1 : CombinatorialLogic  TruthTable=[0 0 0 0 0 0 0 0 0 0 0 0 0 0 0 0; 0 1 0 0 0 0 0 0 0 0 0 0 0 0 0 0]
  Combinatorial Logic10 : CombinatorialLogic  TruthTable=[0 0 0 0 0 0 0 0 0 0 0 0 0 0 0 0;0 0 0 0 0 0 0 0 0 1 0 0 0 0 0 0]
  Combinatorial Logic11 : CombinatorialLogic  TruthTable=[0 0 0 0 0 0 0 0 0 0 0 0 0 0 0 0;0 0 0 0 0 0 0 0 0 0 1 0 0 0 0 0 ]
  Combinatorial Logic12 : CombinatorialLogic  TruthTable=[0 0 0 0 0 0 0 0 0 0 0 0 0 0 0 0;0 0 0 0 0 0 0 0 0 0 0 0 1 0 0 0]
  Combinatorial Logic13 : CombinatorialLogic  TruthTable=[0 0 0 0 0 0 0 0 0 0 0 0 0 0 0 0;0 0 0 0 0 0 0 0 0 0 0 0 0 1 0 0]
  Combinatorial Logic14 : CombinatorialLogic  TruthTable=[0 0 0 0 0 0 0 0 0 0 0 0 0 0 0 0;0 0 0 0 0 0 0 0 0 0 0 0 0 0 1 0]
  Combinatorial Logic15 : CombinatorialLogic  TruthTable=[0 0 0 0 0 0 0 0 0 0 0 0 0 0 0 0;0 0 0 0 0 0 0 0 0 0 0 0 0 0 0 1]
  Combinatorial Logic2 : CombinatorialLogic  TruthTable=[0 0 0 0 0 0 0 0 0 0 0 0 0 0 0 0;0 0 1 0 0 0 0 0 0 0 0 0 0 0 0 0]
  Combinatorial Logic3 : CombinatorialLogic  TruthTable=[0 0 0 0 0 0 0 0 0 0 0 0 0 0 0 0;0 0 0 1 0 0 0 0 0 0 0 0 0 0 0 0]
  Combinatorial Logic4 : CombinatorialLogic  TruthTable=[0 0 0 0 0 0 0 0 0 0 0 0 0 0 0 0;0 0 0 0 1 0 0 0 0 0 0 0 0 0 0 0]
  Combinatorial Logic5 : CombinatorialLogic  TruthTable=[0 0 0 0 0 0 0 0 0 0 0 0 0 0 0 0;0 0 0 0 0 1 0 0 0 0 0 0 0 0 0 0]
  Combinatorial Logic6 : CombinatorialLogic  TruthTable=[0 0 0 0 0 0 0 0 0 0 0 0 0 0 0 0;0 0 0 0 0 0 1 0 0 0 0 0 0 0 0 0]
  Combinatorial Logic7 : CombinatorialLogic  TruthTable=[0 0 0 0 0 0 0 0 0 0 0 0 0 0 0 0;0 0 0 0 0 0 0 1 0 0 0 0 0 0 0 0]
  Combinatorial Logic8 : CombinatorialLogic  TruthTable=[0 0 0 0 0 0 0 0 0 0 0 0 0 0 0 0;0 0 0 0 0 0 0 0 1 0 0 0 0 0 0 0]
  Combinatorial Logic9 : CombinatorialLogic  TruthTable=[0 0 0 0 0 0 0 0 0 0 0 0 0 0 0 0;0 0 0 0 0 0 0 0 0 0 0 1 0 0 0 0 ]
  Compare To Constnt : simulink/Logic and Bit Operations/Compare To Constant  relop===  const=0  OutDataTypeStr=boolean  ZeroCross=off
  Compare To Constnt1 : simulink/Logic and Bit Operations/Compare To Constant  relop===  const=1  OutDataTypeStr=boolean  ZeroCross=off
  Compare To Constnt10 : simulink/Logic and Bit Operations/Compare To Constant  relop===  const=10  OutDataTypeStr=boolean  ZeroCross=off
  Compare To Constnt11 : simulink/Logic and Bit Operations/Compare To Constant  relop===  const=11  OutDataTypeStr=boolean  ZeroCross=off
  Compare To Constnt12 : simulink/Logic and Bit Operations/Compare To Constant  relop===  const=12  OutDataTypeStr=boolean  ZeroCross=off
  Compare To Constnt13 : simulink/Logic and Bit Operations/Compare To Constant  relop===  const=13  OutDataTypeStr=boolean  ZeroCross=off
  Compare To Constnt14 : simulink/Logic and Bit Operations/Compare To Constant  relop===  const=14  OutDataTypeStr=boolean  ZeroCross=off
  Compare To Constnt15 : simulink/Logic and Bit Operations/Compare To Constant  relop===  const=15  OutDataTypeStr=boolean  ZeroCross=off
  Compare To Constnt2 : simulink/Logic and Bit Operations/Compare To Constant  relop===  const=2  OutDataTypeStr=boolean  ZeroCross=off
  Compare To Constnt3 : simulink/Logic and Bit Operations/Compare To Constant  relop===  const=3  OutDataTypeStr=boolean  ZeroCross=off
  Compare To Constnt4 : simulink/Logic and Bit Operations/Compare To Constant  relop===  const=4  OutDataTypeStr=boolean  ZeroCross=off
  Compare To Constnt5 : simulink/Logic and Bit Operations/Compare To Constant  relop===  const=5  OutDataTypeStr=boolean  ZeroCross=off
  Compare To Constnt6 : simulink/Logic and Bit Operations/Compare To Constant  relop===  const=6  OutDataTypeStr=boolean  ZeroCross=off
  Compare To Constnt7 : simulink/Logic and Bit Operations/Compare To Constant  relop===  const=7  OutDataTypeStr=boolean  ZeroCross=off
  Compare To Constnt8 : simulink/Logic and Bit Operations/Compare To Constant  relop===  const=8  OutDataTypeStr=boolean  ZeroCross=off
  Compare To Constnt9 : simulink/Logic and Bit Operations/Compare To Constant  relop===  const=9  OutDataTypeStr=boolean  ZeroCross=off
  Logical Operator : Logic  Operator=OR  Inputs=16  AllPortsSameDT=off  OutDataTypeStr=boolean
  Out1 : Outport
  wires:
  Logical Operator/1 -> Out1/1
  In1/1 -> Compare To Constnt/1, Compare To Constnt1/1, Compare To Constnt2/1, Compare To Constnt3/1, Compare To Constnt4/1, Compare To Constnt5/1, Compare To Constnt6/1, Compare To Constnt7/1, Compare To Constnt8/1, Compare To Constnt9/1, Compare To Constnt10/1, Compare To Constnt11/1, Compare To Constnt12/1, Compare To Constnt13/1, Compare To Constnt15/1, Compare To Constnt14/1
  Compare To Constnt/1 -> Combinatorial Logic/1
  Compare To Constnt1/1 -> Combinatorial Logic1/1
  Compare To Constnt2/1 -> Combinatorial Logic2/1
  Compare To Constnt3/1 -> Combinatorial Logic3/1
  Compare To Constnt4/1 -> Combinatorial Logic4/1
  Compare To Constnt5/1 -> Combinatorial Logic5/1
  Compare To Constnt6/1 -> Combinatorial Logic6/1
  Compare To Constnt7/1 -> Combinatorial Logic7/1
  Combinatorial Logic/1 -> Logical Operator/1
  Combinatorial Logic1/1 -> Logical Operator/2
  Combinatorial Logic2/1 -> Logical Operator/3
  Combinatorial Logic3/1 -> Logical Operator/4
  Combinatorial Logic4/1 -> Logical Operator/5
  Combinatorial Logic5/1 -> Logical Operator/6
  Combinatorial Logic6/1 -> Logical Operator/7
  Combinatorial Logic7/1 -> Logical Operator/8
  Compare To Constnt8/1 -> Combinatorial Logic8/1
  Compare To Constnt9/1 -> Combinatorial Logic10/1
  Compare To Constnt10/1 -> Combinatorial Logic11/1
  Compare To Constnt11/1 -> Combinatorial Logic9/1
  Compare To Constnt12/1 -> Combinatorial Logic12/1
  Compare To Constnt13/1 -> Combinatorial Logic13/1
  Compare To Constnt14/1 -> Combinatorial Logic14/1
  Compare To Constnt15/1 -> Combinatorial Logic15/1
  Combinatorial Logic8/1 -> Logical Operator/9
  Combinatorial Logic10/1 -> Logical Operator/10
  Combinatorial Logic11/1 -> Logical Operator/11
  Combinatorial Logic9/1 -> Logical Operator/12
  Combinatorial Logic12/1 -> Logical Operator/13
  Combinatorial Logic13/1 -> Logical Operator/14
  Combinatorial Logic14/1 -> Logical Operator/15
  Combinatorial Logic15/1 -> Logical Operator/16

== system AVIC_model/2値3次 NSDEM/NSDEM_3rd/SELECTOR1/Subsystem3 ==
  In1 : Inport
  Combinatorial Logic : CombinatorialLogic  TruthTable=[0 0 0 0 0 0 0 0 0 0 0 0 0 0 0 0;1 0 0 0 0 0 0 0 0 0 0 0 0 0 0 0]
  Combinatorial Logic1 : CombinatorialLogic  TruthTable=[0 0 0 0 0 0 0 0 0 0 0 0 0 0 0 0; 0 1 0 0 0 0 0 0 0 0 0 0 0 0 0 0]
  Combinatorial Logic10 : CombinatorialLogic  TruthTable=[0 0 0 0 0 0 0 0 0 0 0 0 0 0 0 0;0 0 0 0 0 0 0 0 0 1 0 0 0 0 0 0]
  Combinatorial Logic11 : CombinatorialLogic  TruthTable=[0 0 0 0 0 0 0 0 0 0 0 0 0 0 0 0;0 0 0 0 0 0 0 0 0 0 1 0 0 0 0 0 ]
  Combinatorial Logic12 : CombinatorialLogic  TruthTable=[0 0 0 0 0 0 0 0 0 0 0 0 0 0 0 0;0 0 0 0 0 0 0 0 0 0 0 0 1 0 0 0]
  Combinatorial Logic13 : CombinatorialLogic  TruthTable=[0 0 0 0 0 0 0 0 0 0 0 0 0 0 0 0;0 0 0 0 0 0 0 0 0 0 0 0 0 1 0 0]
  Combinatorial Logic14 : CombinatorialLogic  TruthTable=[0 0 0 0 0 0 0 0 0 0 0 0 0 0 0 0;0 0 0 0 0 0 0 0 0 0 0 0 0 0 1 0]
  Combinatorial Logic15 : CombinatorialLogic  TruthTable=[0 0 0 0 0 0 0 0 0 0 0 0 0 0 0 0;0 0 0 0 0 0 0 0 0 0 0 0 0 0 0 1]
  Combinatorial Logic2 : CombinatorialLogic  TruthTable=[0 0 0 0 0 0 0 0 0 0 0 0 0 0 0 0;0 0 1 0 0 0 0 0 0 0 0 0 0 0 0 0]
  Combinatorial Logic3 : CombinatorialLogic  TruthTable=[0 0 0 0 0 0 0 0 0 0 0 0 0 0 0 0;0 0 0 1 0 0 0 0 0 0 0 0 0 0 0 0]
  Combinatorial Logic4 : CombinatorialLogic  TruthTable=[0 0 0 0 0 0 0 0 0 0 0 0 0 0 0 0;0 0 0 0 1 0 0 0 0 0 0 0 0 0 0 0]
  Combinatorial Logic5 : CombinatorialLogic  TruthTable=[0 0 0 0 0 0 0 0 0 0 0 0 0 0 0 0;0 0 0 0 0 1 0 0 0 0 0 0 0 0 0 0]
  Combinatorial Logic6 : CombinatorialLogic  TruthTable=[0 0 0 0 0 0 0 0 0 0 0 0 0 0 0 0;0 0 0 0 0 0 1 0 0 0 0 0 0 0 0 0]
  Combinatorial Logic7 : CombinatorialLogic  TruthTable=[0 0 0 0 0 0 0 0 0 0 0 0 0 0 0 0;0 0 0 0 0 0 0 1 0 0 0 0 0 0 0 0]
  Combinatorial Logic8 : CombinatorialLogic  TruthTable=[0 0 0 0 0 0 0 0 0 0 0 0 0 0 0 0;0 0 0 0 0 0 0 0 1 0 0 0 0 0 0 0]
  Combinatorial Logic9 : CombinatorialLogic  TruthTable=[0 0 0 0 0 0 0 0 0 0 0 0 0 0 0 0;0 0 0 0 0 0 0 0 0 0 0 1 0 0 0 0 ]
  Compare To Constnt : simulink/Logic and Bit Operations/Compare To Constant  relop===  const=0  OutDataTypeStr=boolean  ZeroCross=off
  Compare To Constnt1 : simulink/Logic and Bit Operations/Compare To Constant  relop===  const=1  OutDataTypeStr=boolean  ZeroCross=off
  Compare To Constnt10 : simulink/Logic and Bit Operations/Compare To Constant  relop===  const=10  OutDataTypeStr=boolean  ZeroCross=off
  Compare To Constnt11 : simulink/Logic and Bit Operations/Compare To Constant  relop===  const=11  OutDataTypeStr=boolean  ZeroCross=off
  Compare To Constnt12 : simulink/Logic and Bit Operations/Compare To Constant  relop===  const=12  OutDataTypeStr=boolean  ZeroCross=off
  Compare To Constnt13 : simulink/Logic and Bit Operations/Compare To Constant  relop===  const=13  OutDataTypeStr=boolean  ZeroCross=off
  Compare To Constnt14 : simulink/Logic and Bit Operations/Compare To Constant  relop===  const=14  OutDataTypeStr=boolean  ZeroCross=off
  Compare To Constnt15 : simulink/Logic and Bit Operations/Compare To Constant  relop===  const=15  OutDataTypeStr=boolean  ZeroCross=off
  Compare To Constnt2 : simulink/Logic and Bit Operations/Compare To Constant  relop===  const=2  OutDataTypeStr=boolean  ZeroCross=off
  Compare To Constnt3 : simulink/Logic and Bit Operations/Compare To Constant  relop===  const=3  OutDataTypeStr=boolean  ZeroCross=off
  Compare To Constnt4 : simulink/Logic and Bit Operations/Compare To Constant  relop===  const=4  OutDataTypeStr=boolean  ZeroCross=off
  Compare To Constnt5 : simulink/Logic and Bit Operations/Compare To Constant  relop===  const=5  OutDataTypeStr=boolean  ZeroCross=off
  Compare To Constnt6 : simulink/Logic and Bit Operations/Compare To Constant  relop===  const=6  OutDataTypeStr=boolean  ZeroCross=off
  Compare To Constnt7 : simulink/Logic and Bit Operations/Compare To Constant  relop===  const=7  OutDataTypeStr=boolean  ZeroCross=off
  Compare To Constnt8 : simulink/Logic and Bit Operations/Compare To Constant  relop===  const=8  OutDataTypeStr=boolean  ZeroCross=off
  Compare To Constnt9 : simulink/Logic and Bit Operations/Compare To Constant  relop===  const=9  OutDataTypeStr=boolean  ZeroCross=off
  Logical Operator : Logic  Operator=OR  Inputs=16  AllPortsSameDT=off  OutDataTypeStr=boolean
  Out1 : Outport
  wires:
  Logical Operator/1 -> Out1/1
  In1/1 -> Compare To Constnt/1, Compare To Constnt1/1, Compare To Constnt2/1, Compare To Constnt3/1, Compare To Constnt4/1, Compare To Constnt5/1, Compare To Constnt6/1, Compare To Constnt7/1, Compare To Constnt8/1, Compare To Constnt9/1, Compare To Constnt10/1, Compare To Constnt11/1, Compare To Constnt12/1, Compare To Constnt13/1, Compare To Constnt15/1, Compare To Constnt14/1
  Compare To Constnt/1 -> Combinatorial Logic/1
  Compare To Constnt1/1 -> Combinatorial Logic1/1
  Compare To Constnt2/1 -> Combinatorial Logic2/1
  Compare To Constnt3/1 -> Combinatorial Logic3/1
  Compare To Constnt4/1 -> Combinatorial Logic4/1
  Compare To Constnt5/1 -> Combinatorial Logic5/1
  Compare To Constnt6/1 -> Combinatorial Logic6/1
  Compare To Constnt7/1 -> Combinatorial Logic7/1
  Combinatorial Logic/1 -> Logical Operator/1
  Combinatorial Logic1/1 -> Logical Operator/2
  Combinatorial Logic2/1 -> Logical Operator/3
  Combinatorial Logic3/1 -> Logical Operator/4
  Combinatorial Logic4/1 -> Logical Operator/5
  Combinatorial Logic5/1 -> Logical Operator/6
  Combinatorial Logic6/1 -> Logical Operator/7
  Combinatorial Logic7/1 -> Logical Operator/8
  Compare To Constnt8/1 -> Combinatorial Logic8/1
  Compare To Constnt9/1 -> Combinatorial Logic10/1
  Compare To Constnt10/1 -> Combinatorial Logic11/1
  Compare To Constnt11/1 -> Combinatorial Logic9/1
  Compare To Constnt12/1 -> Combinatorial Logic12/1
  Compare To Constnt13/1 -> Combinatorial Logic13/1
  Compare To Constnt14/1 -> Combinatorial Logic14/1
  Compare To Constnt15/1 -> Combinatorial Logic15/1
  Combinatorial Logic8/1 -> Logical Operator/9
  Combinatorial Logic10/1 -> Logical Operator/10
  Combinatorial Logic11/1 -> Logical Operator/11
  Combinatorial Logic9/1 -> Logical Operator/12
  Combinatorial Logic12/1 -> Logical Operator/13
  Combinatorial Logic13/1 -> Logical Operator/14
  Combinatorial Logic14/1 -> Logical Operator/15
  Combinatorial Logic15/1 -> Logical Operator/16
